simulink model "massignment6"  (Simulink 6.0)
settings: Solver=FixedStepDiscrete  StartTime=0.0  StopTime=10.0  RelTol=1e-3
libraries: massignmentLib x2
settings Model: Creator=awarlock  LastModifiedBy=byu  ExtModeAutoUpdateStatusClock=off
settings OptimizationCC: InlineParams=on
settings DebuggingCC: SolverPrmCheckMsg=none  MultiTaskDSMMsg=warning

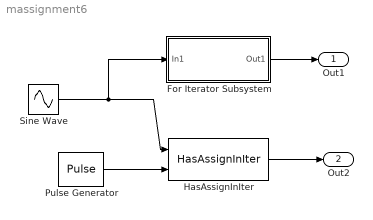
== system massignment6 ==
  For Iterator Subsystem : Subsystem  TreatAsAtomicUnit=on
  HasAssignInIter : massignmentLib/HasAssignInIter
  Pulse Generator : DiscretePulseGenerator  SampleTime=0.1
  Sine Wave : Sin  Amplitude=3:7  SampleTime=0.1
  Out1 : Outport
  Out2 : Outport  Port=2
  wires:
  Sine Wave/1 -> For Iterator Subsystem/1(In1), HasAssignInIter/1
  For Iterator Subsystem/1(Out1) -> Out1/1
  HasAssignInIter/1 -> Out2/1
  Pulse Generator/1 -> HasAssignInIter/2

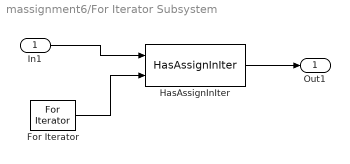
== system massignment6/For Iterator Subsystem ==
  In1 : Inport  Port=1  LatchInput=off
  For Iterator : ForIterator  IterationVariableDataType=double
  HasAssignInIter : massignmentLib/HasAssignInIter
  Out1 : Outport
  wires:
  In1/1 -> HasAssignInIter/1
  For Iterator/1 -> HasAssignInIter/2
  HasAssignInIter/1 -> Out1/1
